simulink model "Control_model_10DOF_fin"  (R2016b)
settings: Solver=FixedStepAuto  StartTime=0.0  StopTime=10  FixedStep=0.0001  RelTol=1e-3
InitFcn:
  | Initialisation_ctr_10DOF_fin
values from neighbouring files (symbols this model uses):
  COM_Parameters = [-lpelvis/2;r2;0]    [Initialisation_ctr_10DOF_fin.m]
  DH_Parameters = [hfoot 0 ... (first row only)    [Initialisation_ctr_10DOF_fin.m]
  dTrunk = trunklbd(3)    [Initialisation_ctr_10DOF_fin.m]
  dxFootSM = dxFoot    [Initialisation_ctr_10DOF_fin.m]
  dxTrunk = 0.1    [Initialisation_ctr_10DOF_fin.m]
  Foot_Parameters = [0;-(lFoot/2-lHeel);0]    [Initialisation_ctr_10DOF_fin.m]
  HAA2HEE = [0; 0; 0.001]    [Initialisation_ctr_10DOF_fin.m]
  HEE2HFE = 0.5*[0.2; 0; 0]    [Initialisation_ctr_10DOF_fin.m]
  height_vrp = CoM_position(1)    [Initialisation_ctr_10DOF_fin.m]
  hTrunk = trunklbd(1)    [Initialisation_ctr_10DOF_fin.m]
  initial_CoM_position = R*CoM_position    [Initialisation_ctr_10DOF_fin.m]
  initial_CoM_velocity = [0;0;0]    [Initialisation_ctr_10DOF_fin.m]
  initial_left_foot = [0;0;-stance_width/2]    [Initialisation_ctr_10DOF_fin.m]
  initial_right_foot = [0;0;stance_width/2]    [Initialisation_ctr_10DOF_fin.m]
  initial_RorL = 0    [Initialisation_ctr_10DOF_fin.m]
  jointsinitial = [9;-15;6;0;0;6;-15;9]/180*pi    [Initialisation_ctr_10DOF_fin.m]
  K_DCM = 4.3*[1 0 0 ... (first row only)    [Initialisation_ctr_10DOF_fin.m]
  kD_left = mbody*[0.95 0 0 0 ... (first row only)    [Initialisation_ctr_10DOF_fin.m]
  kD_right = mbody*[0.12 0 0 0 ... (first row only)    [Initialisation_ctr_10DOF_fin.m]
  kI_left = mbody*[35 0 0 0 ... (first row only)    [Initialisation_ctr_10DOF_fin.m]
  kI_right = mbody*[38.2 0 0 0 ... (first row only)    [Initialisation_ctr_10DOF_fin.m]
  kP_left = mbody*[75 0 0 0 ... (first row only)    [Initialisation_ctr_10DOF_fin.m]
  kP_right = mbody*[5.6 0 0 0 ... (first row only)    [Initialisation_ctr_10DOF_fin.m]
  Lenght = [lShank;lThigh]    [Initialisation_ctr_10DOF_fin.m]
  lFootSM = lFoot    [Initialisation_ctr_10DOF_fin.m]
  lpelvis = wPelvis    [Initialisation_ctr_10DOF_fin.m]
  mass = mbody    (= 60)    [Initialisation_ctr_10DOF_fin.m]
  Masses = [mThigh; mShank; mTrunk]    [Initialisation_ctr_10DOF_fin.m]
  nb_step = 4    [Initialisation_ctr_10DOF_fin.m]
  nb_step_pattern = 20    [Initialisation_ctr_10DOF_fin.m]
  Pelvis_Parameters = [-lpelvis/2;hTrunk/2;0]    [Initialisation_ctr_10DOF_fin.m]
  stance_width = lpelvis    [Initialisation_ctr_10DOF_fin.m]
  stride_lenght = 0.50    (= 0.5)    [Initialisation_ctr_10DOF_fin.m]
  T_DS = time_DS    (= 0.4)    [Initialisation_ctr_10DOF_fin.m]
  T_IT = time_DS    (= 0.4)    [Initialisation_ctr_10DOF_fin.m]
  T_SS = time_swing    (= 1.6)    [Initialisation_ctr_10DOF_fin.m]
  time_DS = (time_stance-time_swing)/2    (= 0.4)    [Initialisation_ctr_10DOF_fin.m]
  time_stance = 60/100*time_stride    (= 2.4)    [Initialisation_ctr_10DOF_fin.m]
  time_step = time_stride/2    (= 2)    [Initialisation_ctr_10DOF_fin.m]
  time_swing = 40/100*time_stride    (= 1.6)    [Initialisation_ctr_10DOF_fin.m]
  validity_angle = [-20*pi/180 20*pi/180 ... (first row only)    [Initialisation_ctr_10DOF_fin.m]
  wTrunk = trunklbd(2)    [Initialisation_ctr_10DOF_fin.m]
  x4CoM = CoM_position(1)-XR4(1)    [Initialisation_ctr_10DOF_fin.m]
undefined symbols (not defined in the file or in its folder): dsegment, hFoot, l, lFoot, omega0_x, omega0_z, rho, wPelvis, X, Xp_x, Xp_z, Y, Z
undefined symbols (not defined in the file): k_grf, lShankSM, lThighSM, mShank, mThigh
libraries: nesl_utility x247, sm_lib x215, dspindex x12, FootPlacementLibrary x8, dspsigops x4, dspswit3 x1
(part 13 of 18)

== matlab function Control_model_10DOF_fin/10DoF Walker SimMechanics Model/Foot/GRF2 Toe/MATLAB Function1 ==
  data: x input; dx input; y input; dy input; z input; Fx output; dz input; Fy output; k input; Fz output
function [Fx,Fy,Fz]= fcn(x,dx,y,dy,z,dz,k)
%#codegen
% k=[5*10^4 10^4 0 10^4 0];
%k=[5*10^4 10^4 0 0 0];
% k=[0 0 0 0 0];

kp = k(1);
kv = k(2);
kpt = k(3);
kvt = k(4);
mu = k(5);

persistent prevContact;

if y>0
    Fy = 0;
    Fxz = [0;0];
    prevContact = [];
else
    if isempty(prevContact)
        prevContact = [x;z];
    end
    Current = [x;z];
    
    Fy = -kp*y-kv*dy;
%     Fxz = -kpt*(Current-prevContact)-kvt*[dx;dz];
    Fxz = -kvt*[dx;dz];
end

if Fy<0;
    Fy = 0;
%     prevContact = [];
end

mu=1;
if norm(Fxz)>mu*norm(Fy)
    Fxz = Fxz/norm(Fxz)*mu*norm(Fy);
end

Fx = Fxz(1);
Fz = Fxz(2);

== matlab function Control_model_10DOF_fin/10DoF Walker SimMechanics Model/Foot/MATLAB Function ==
  data: R_foot_pos input; TW0 output; R_foot_Rotation input; XWankleR output; Foot_Parameters parameter; DH_Parameters parameter
function [TW0,XWankleR] = fcn(R_foot_pos,R_foot_Rotation,Foot_Parameters,DH_Parameters)

% TWR=[R_foot_Rotation(1,2) R_foot_Rotation(1,1) -R_foot_Rotation(1,3) R_foot_pos(2);
%     R_foot_Rotation(2,2) R_foot_Rotation(2,1) -R_foot_Rotation(2,3) R_foot_pos(1);
%     R_foot_Rotation(3,2) R_foot_Rotation(3,1) -R_foot_Rotation(3,3) -R_foot_pos(3)
%     0 0 0 1];

xfoot=Foot_Parameters(1);
yfoot=Foot_Parameters(2);
zfoot=Foot_Parameters(3);

a0=DH_Parameters(1,1);
d1=DH_Parameters(1,2);
a1=DH_Parameters(2,1);
d2=DH_Parameters(2,2);
a2=DH_Parameters(3,1);
d3=DH_Parameters(3,2);
a3=DH_Parameters(4,1);
d4=DH_Parameters(4,2);
a4=DH_Parameters(5,1);
d5=DH_Parameters(5,2);
a5=DH_Parameters(6,1);
d6=DH_Parameters(6,2);
a6=DH_Parameters(7,1);
d7=DH_Parameters(7,2);
a7=DH_Parameters(8,1);
d8=DH_Parameters(8,2);
a8=DH_Parameters(9,1);
d9=DH_Parameters(9,2);

TWR_D=[R_foot_Rotation(1,1) R_foot_Rotation(1,2) R_foot_Rotation(1,3) R_foot_pos(1);
    R_foot_Rotation(2,1) R_foot_Rotation(2,2) R_foot_Rotation(2,3) R_foot_pos(2);
    R_foot_Rotation(3,1) R_foot_Rotation(3,2) R_foot_Rotation(3,3) R_foot_pos(3);
    0 0 0 1];

T=[0 1 0 0;
    1 0 0 0;
    0 0 -1 0;
    0 0 0 1];

TWR=TWR_D*T;

TR0=[1 0 0 xfoot;
    0 1 0 yfoot;
    0 0 1 zfoot;
    0 0 0 1];

T0ankleR=[1 0 0 a0;
    0 1 0 0;
    0 0 1 0;
    0 0 0 1];

TW0=TWR*TR0;
TWankleR=TW0*T0ankleR;

XWR=TWR(1:3,4);
XW0=TW0(1:3,4);
XWankleR=TWankleR(1:3,4);

== matlab function Control_model_10DOF_fin/10DoF Walker SimMechanics Model/Foot1/GRF1 Heel/MATLAB Function1 ==
  data: x input; dx input; y input; dy input; z input; Fx output; dz input; Fy output; k input; Fz output
function [Fx,Fy,Fz]= fcn(x,dx,y,dy,z,dz,k)
%#codegen
% k=[5*10^4 10^4 0 10^4 0];
% k=[5*10^4 10^4 0 0 0];
% k=[0 0 0 0 0];

kp = k(1);
kv = k(2);
kpt = k(3);
kvt = k(4);
mu = k(5);

persistent prevContact;

if y>0
    Fy = 0;
    Fxz = [0;0];
    prevContact = [];
else
    if isempty(prevContact)
        prevContact = [x;z];
    end
    Current = [x;z];
    
    Fy = -kp*y-kv*dy;
%     Fxz = -kpt*(Current-prevContact)-kvt*[dx;dz];
    Fxz = -kvt*[dx;dz];
end

if Fy<0
    Fy = 0;
%     prevContact = [];
end

mu=1;
if norm(Fxz)>mu*norm(Fy)
    Fxz = Fxz/norm(Fxz)*mu*norm(Fy);
end

Fx = Fxz(1);
Fz = Fxz(2);

== matlab function Control_model_10DOF_fin/10DoF Walker SimMechanics Model/Foot1/GRF1 Toe/MATLAB Function1 ==
  data: x input; dx input; y input; dy input; z input; Fx output; dz input; Fy output; k input; Fz output
function [Fx,Fy,Fz]= fcn(x,dx,y,dy,z,dz,k)
%#codegen
% k=[5*10^4 10^4 0 10^4 0];
%k=[5*10^4 10^4 0 0 0];
% k=[0 0 0 0 0];

kp = k(1);
kv = k(2);
kpt = k(3);
kvt = k(4);
mu = k(5);

persistent prevContact;

if y>0
    Fy = 0;
    Fxz = [0;0];
    prevContact = [];
else
    if isempty(prevContact)
        prevContact = [x;z];
    end
    Current = [x;z];
    
    Fy = -kp*y-kv*dy;
%     Fxz = -kpt*(Current-prevContact)-kvt*[dx;dz];
    Fxz = -kvt*[dx;dz];
end

if Fy<0;
    Fy = 0;
%     prevContact = [];
end

mu=1;
if norm(Fxz)>mu*norm(Fy)
    Fxz = Fxz/norm(Fxz)*mu*norm(Fy);
end

Fx = Fxz(1);
Fz = Fxz(2);

== matlab function Control_model_10DOF_fin/10DoF Walker SimMechanics Model/Foot1/GRF2 Heel/MATLAB Function1 ==
  data: x input; dx input; y input; dy input; z input; Fx output; dz input; Fy output; k input; Fz output
function [Fx,Fy,Fz]= fcn(x,dx,y,dy,z,dz,k)
%#codegen
% k=[5*10^4 10^4 0 10^4 0];
% k=[5*10^4 10^4 0 0 0];
% k=[0 0 0 0 0];

kp = k(1);
kv = k(2);
kpt = k(3);
kvt = k(4);
mu = k(5);

persistent prevContact;

if y>0
    Fy = 0;
    Fxz = [0;0];
    prevContact = [];
else
    if isempty(prevContact)
        prevContact = [x;z];
    end
    Current = [x;z];
    
    Fy = -kp*y-kv*dy;
%     Fxz = -kpt*(Current-prevContact)-kvt*[dx;dz];
    Fxz = -kvt*[dx;dz];
end

if Fy<0
    Fy = 0;
%     prevContact = [];
end

mu=1;
if norm(Fxz)>mu*norm(Fy)
    Fxz = Fxz/norm(Fxz)*mu*norm(Fy);
end

Fx = Fxz(1);
Fz = Fxz(2);

== matlab function Control_model_10DOF_fin/10DoF Walker SimMechanics Model/Foot1/GRF2 Toe/MATLAB Function1 ==
  data: x input; dx input; y input; dy input; z input; Fx output; dz input; Fy output; k input; Fz output
function [Fx,Fy,Fz]= fcn(x,dx,y,dy,z,dz,k)
%#codegen
% k=[5*10^4 10^4 0 10^4 0];
%k=[5*10^4 10^4 0 0 0];
% k=[0 0 0 0 0];

kp = k(1);
kv = k(2);
kpt = k(3);
kvt = k(4);
mu = k(5);

persistent prevContact;

if y>0
    Fy = 0;
    Fxz = [0;0];
    prevContact = [];
else
    if isempty(prevContact)
        prevContact = [x;z];
    end
    Current = [x;z];
    
    Fy = -kp*y-kv*dy;
%     Fxz = -kpt*(Current-prevContact)-kvt*[dx;dz];
    Fxz = -kvt*[dx;dz];
end

if Fy<0
    Fy = 0;
%     prevContact = [];
end

mu=1;
if norm(Fxz)>mu*norm(Fy)
    Fxz = Fxz/norm(Fxz)*mu*norm(Fy);
end

Fx = Fxz(1);
Fz = Fxz(2);

== matlab function Control_model_10DOF_fin/10DoF Walker SimMechanics Model/Graphic/Joint position/T->X/MATLAB Function ==
  data: XWR output; XW0 output; TWR input; TW0 input; TW1 input; XW1 output; TW2 input; TW3 input; XW2 output; TW4 input; TW5 input; TW6 input; TW7 input; TW8 input; TW9 input; TWL input; XW3 output; XW4 output; XW5 output; XW6 output; XW7 output; XW8 output; XWcom input; XW9 output; XWL output; TWthighR input; XWCoM output; TWshankR input; TWtrunk input; TWshankL input; TWthighL input; XWthighR output; XWthighL output; XWshankR output; XWshankL output; XWtrunk output
function [XWR,XW0,XW1,XW2,XW3,XW4,XW5,XW6,XW7,XW8,XW9,XWL,XWCoM,XWthighR,XWthighL,XWshankR,XWshankL,XWtrunk] = Joint_position(TWR,TW0,TW1,TW2,TW3,TW4,TW5,TW6,TW7,TW8,TW9,TWL,XWcom,TWthighR,TWshankR,TWtrunk,TWshankL,TWthighL)

XWR=TWR(1:3,4);
XW0=TW0(1:3,4);
XW1=TW1(1:3,4);
XW2=TW2(1:3,4);
XW3=TW3(1:3,4);
XW4=TW4(1:3,4);
XW5=TW5(1:3,4);
XW6=TW6(1:3,4);
XW7=TW7(1:3,4);
XW8=TW8(1:3,4);
XW9=TW9(1:3,4);
XWL=TWL(1:3,4);
XWCoM=XWcom;
XWthighR=TWthighR(1:3,4);
XWthighL=TWthighL(1:3,4);
XWshankR=TWshankR(1:3,4);
XWshankL=TWshankL(1:3,4);
XWtrunk=TWtrunk(1:3,4);

== matlab function Control_model_10DOF_fin/10DoF Walker SimMechanics Model/Graphic/Subsystem/MATLAB Function1 ==
  data: Right_foot_position input; R1 output; Left_foot_position input; lFoot parameter; dsegment parameter; r_vrp input size=3; r_DCM input size=3; R2 output; R3 output; R4 output; L1 output; L2 output; L3 output; L4 output; new_vrp output; outside output
function [R1,R2,R3,R4,L1,L2,L3,L4,new_vrp,outside] = support_polygon(Right_foot_position,Left_foot_position,lFoot,dsegment,r_vrp,r_DCM)
R1=Right_foot_position+[0;lFoot/2;dsegment/2];
R2=Right_foot_position+[0;lFoot/2;-dsegment/2];
R3=Right_foot_position+[0;-lFoot/2;-dsegment/2];
R4=Right_foot_position+[0;-lFoot/2;dsegment/2];

L1=Left_foot_position+[0;lFoot/2;dsegment/2];
L2=Left_foot_position+[0;lFoot/2;-dsegment/2];
L3=Left_foot_position+[0;-lFoot/2;-dsegment/2];
L4=Left_foot_position+[0;-lFoot/2;dsegment/2];

%Calcul affine line
a1=(L4(2)-R4(2))/(L4(3)-R4(3));
b1=R4(2)-a1*R4(3);

a2=(L2(2)-R2(2))/(L2(3)-R2(3));
b2=R2(2)-a2*R2(3);

a3=(r_vrp(2)-r_DCM(2))/(r_vrp(3)-r_DCM(3));
b3=r_DCM(2)-a3*r_DCM(3);

%Check if outside support polygon (1=outside,0=indside)
outside=0;



if ((r_vrp(2)<R3(2)) || (r_vrp(2)>L1(2)) || (r_vrp(3)<R3(3)) || (r_vrp(3)>L1(3)))
    outside=1;
elseif (r_vrp(2)<a1*r_vrp(3)+b1) || (r_vrp(2)>a2*r_vrp(3)+b2)
        outside=1;
end

% if outside ==1
% else
%     new_vrp=r_vrp;
% end


new_vrp=r_vrp;
if outside==1
    if r_vrp(3)<=R3(3)
        new_vrp(3)=R3(3);
        new_vrp(2)=a3*new_vrp(3)+b3;
        if new_vrp(2)<R3(2)
            new_vrp(2)=R3(2);
            new_vrp(3)=(new_vrp(2)-b3)/a3;
            if new_vrp(3)<R3(3)
                new_vrp(2)=R3(2);
                new_vrp(3)=R3(3);
            elseif new_vrp(2)<R4(2)
                new_vrp(2)=R4(2);
                new_vrp(3)=R4(3);
            end      
        elseif new_vrp(2)>R2(2)
            new_vrp(3)=(b2-b1)/(a1-a2);
            new_vrp(2)=a3*new_vrp(3)+b3;
            if new_vrp(3)<R2(3)
                new_vrp(2)=R2(2);
                new_vrp(3)=R2(3);
            end
        end
    elseif r_vrp(3)>=L1(3)
        new_vrp(3)=L1(3);
        new_vrp(2)=a3*new_vrp(3)+b3;
        if new_vrp(2)<L4(2)
            new_vrp(3)=(b3-b1)/(a3-a1);
            new_vrp(2)=a3*new_vrp(3)+b3;
            if new_vrp(2)<L4(2)
                new_vrp(2)=L4(2);
                new_vrp(3)=L4(3);
            end
        elseif new_vrp(2)>L1(2)
            new_vrp(2)=L1(2);
            new_vrp(3)=(new_vrp(2)-b3)/a3;
            if new_vrp(3)>L1(3)
                new_vrp(2)=L1(2);
                new_vrp(3)=L1(3);
            elseif new_vrp(3)<L2(3)
                new_vrp(2)=L2(2);
                new_vrp(3)=L2(3);
            end
                
        end
        
    elseif r_vrp(2)<=R3(2)
        new_vrp(2)=R3(2);
        new_vrp(3)=(new_vrp(2)-b3)/a3;
        if new_vrp(3)<R3(3)
            new_vrp(2)=R3(2);
            new_vrp(3)=R3(3);
        elseif new_vrp(3)>R4(3)
                new_vrp(3)=(b3-b1)/(a3-a1);
                new_vrp(2)=a3*new_vrp(3)+b3;
                if new_vrp(3)<R4(3)
                    new_vrp(2)=R4(2);
                    new_vrp(3)=R4(3);
                elseif new_vrp(3)>L4(3)
                    new_vrp(2)=L4(2);
                    new_vrp(3)=L4(3);
                end
        end
    elseif r_vrp(2)>=L1(2)
        new_vrp(2)=L1(2);
        new_vrp(3)=(new_vrp(2)-b3)/a3;
        if new_vrp(3)>L1(3)
            new_vrp(2)=L1(2);
            new_vrp(3)=L1(3);
        elseif new_vrp(3)<L2(3)
            new_vrp(3)=(b2-b3)/(a2-a3);
            new_vrp(2)=a3*new_vrp(3)+b3;
            if new_vrp(3)>L2(3)
                new_vrp(2)=L2(2);
                new_vrp(3)=L2(3);
            elseif new_vrp(3)<R2(3)
                new_vrp(2)=R2(2);
                new_vrp(3)=R3(2);
            end
        end
    end
end

== matlab function Control_model_10DOF_fin/10DoF Walker SimMechanics Model/Graphic/Subsystem/MATLAB Function2 ==
  data: Right_foot_position input; R1 output; Left_foot_position input; lFoot parameter; dsegment parameter; r_vrp input size=3; r_DCM input size=3; R2 output; R3 output; R4 output; L1 output; L2 output; L3 output; L4 output; new_vrp output; outside output; cas output
function [R1,R2,R3,R4,L1,L2,L3,L4,new_vrp,outside,cas] = support_polygon(Right_foot_position,Left_foot_position,lFoot,dsegment,r_vrp,r_DCM)
R1=Right_foot_position+[0;lFoot/2;dsegment/2];
R2=Right_foot_position+[0;lFoot/2;-dsegment/2];
R3=Right_foot_position+[0;-lFoot/2;-dsegment/2];
R4=Right_foot_position+[0;-lFoot/2;dsegment/2];

L1=Left_foot_position+[0;lFoot/2;dsegment/2];
L2=Left_foot_position+[0;lFoot/2;-dsegment/2];
L3=Left_foot_position+[0;-lFoot/2;-dsegment/2];
L4=Left_foot_position+[0;-lFoot/2;dsegment/2];

%Calcul affine line

a1=(L1(2)-R1(2))/(L1(3)-R1(3));
b1=R1(2)-a1*R1(3);

a2=(L2(2)-R2(2))/(L2(3)-R2(3));
b2=R2(2)-a2*R2(3);

a3=(L3(2)-R3(2))/(L3(3)-R3(3));
b3=R3(2)-a3*R3(3);

a4=(L4(2)-R4(2))/(L4(3)-R4(3));
b4=R4(2)-a4*R4(3);

a5=(r_vrp(2)-r_DCM(2))/(r_vrp(3)-r_DCM(3));
b5=r_DCM(2)-a5*r_DCM(3);


%Check if outside support polygon (1=outside,0=indside)
outside=0;






% if outside ==1
% else
%     new_vrp=r_vrp;
% end

point=r_vrp;
point(3)=(b5-b4)/(a5-a4);
point(2)=a5*r_vrp(3)+b5;

cas=0;

new_vrp=r_vrp;

%% Right

if ((r_vrp(2)<R3(2)) || (r_vrp(2)>L1(2)) || (r_vrp(3)<R3(3)) || (r_vrp(3)>L1(3)))
    outside=1;
elseif (r_vrp(2)<a4*r_vrp(3)+b4) || (r_vrp(2)>a2*r_vrp(3)+b2)
        outside=1;
end

if outside==1
    if r_vrp(3)<=R3(3)
        new_vrp(3)=R3(3);
        new_vrp(2)=a5*new_vrp(3)+b5;
        cas=1;
        if new_vrp(2)<R3(2)
            new_vrp(2)=R3(2);
            new_vrp(3)=(new_vrp(2)-b5)/a5;
            cas=2;
            if new_vrp(3)<R3(3)
                new_vrp(2)=R3(2);
                new_vrp(3)=R3(3);
                cas=3;
            elseif new_vrp(2)<R4(2)
                new_vrp(2)=R4(2);
                new_vrp(3)=R4(3);
                cas=4;
            end      
        elseif new_vrp(2)>R2(2)
            new_vrp(3)=(b2-b5)/(a5-a2);
            new_vrp(2)=a5*new_vrp(3)+b5;
            cas=5;
            if new_vrp(3)<R2(3)
                new_vrp(2)=R2(2);
                new_vrp(3)=R2(3);
                cas=6;
            end
        end
    elseif r_vrp(3)>=L1(3)
        new_vrp(3)=L1(3);
        new_vrp(2)=a5*new_vrp(3)+b5;
        cas=7;
        if new_vrp(2)<L4(2)
            new_vrp(3)=(b5-b4)/(a4-a5);
            new_vrp(2)=a5*new_vrp(3)+b5;
            cas=8;
            if new_vrp(3)>L4(3)
                new_vrp(2)=L4(2);
                new_vrp(3)=L4(3);
                cas=9;
            elseif new_vrp(3)<R4(3)
                new_vrp(2)=R4(2);
                new_vrp(3)=R4(3);
                cas=10;
            end
        elseif new_vrp(2)>L1(2)
            new_vrp(2)=L1(2);
            new_vrp(3)=(new_vrp(2)-b5)/a5;
            cas=11;
            if new_vrp(3)>L1(3)
                new_vrp(2)=L1(2);
                new_vrp(3)=L1(3);
                cas=12;
            elseif new_vrp(3)<L2(3)
                new_vrp(2)=L2(2);
                new_vrp(3)=L2(3);
                cas=13;
            end
                
        end
        
    elseif r_vrp(2)<=R3(2)
        new_vrp(2)=R3(2);
        new_vrp(3)=(new_vrp(2)-b5)/a5;
        cas=14;
        if new_vrp(3)<R3(3)
            new_vrp(2)=R3(2);
            new_vrp(3)=R3(3);
            cas=15;
        elseif new_vrp(3)>R4(3)
                new_vrp(3)=(b5-b4)/(a4-a5);
                new_vrp(2)=a5*new_vrp(3)+b5;
                cas=16;
                if new_vrp(3)<R4(3)
                    new_vrp(2)=R4(2);
                    new_vrp(3)=R4(3);
                    cas=17;
                elseif new_vrp(3)>L4(3)
                    new_vrp(2)=L4(2);
                    new_vrp(3)=L4(3);
                    cas=18;
                end
        end
    elseif r_vrp(2)>=L1(2)
        new_vrp(2)=L1(2);
        new_vrp(3)=(new_vrp(2)-b5)/a5;
        cas=19;
        if new_vrp(3)>L1(3)
            new_vrp(2)=L1(2);
            new_vrp(3)=L1(3);
            cas=20;
        elseif new_vrp(3)<L2(3)
            new_vrp(3)=(b2-b5)/(a5-a2);
            new_vrp(2)=a5*new_vrp(3)+b5;
            cas=21;
            if new_vrp(3)>L2(3)
                new_vrp(2)=L2(2);
                new_vrp(3)=L2(3);
                cas=22;
            elseif new_vrp(3)<R2(3)
                new_vrp(2)=R2(2);
                new_vrp(3)=R3(2);
                cas=23;
            end
        end
    elseif (r_vrp(2)<a4*r_vrp(3)+b4)
        new_vrp(3)=(b4-b5)/(a5-a4);
        new_vrp(2)=a5*new_vrp(3)+b5;
        cas=24;
        if new_vrp(3)<R4(3)
            new_vrp(2)=R4(2);
            new_vrp(3)=R4(3);
            cas=25;
        elseif new_vrp(2)>L4
            new_vrp(2)=L4(2);
            new_vrp(3)=L4(3);
            cas=26;
        end
    elseif (r_vrp(2)>a2*r_vrp(3)+b2)
        new_vrp(3)=(b5-b2)/(a2-a5);
        new_vrp(2)=a5*new_vrp(3)+b5;
        cas=27;
        if new_vrp(3)<R2(3)
            new_vrp(2)=R2(2);
            new_vrp(3)=R2(3);
            cas=28;
        elseif new_vrp(3)>L2(3)
            new_vrp(2)=L2(3);
            new_vrp(3)=L2(3);
            cas=29;
        end
    end
end

%% Left

% if ((r_vrp(2)<L4(2)) || (r_vrp(2)>R2(2)) || (r_vrp(3)<R2(3)) || (r_vrp(3)>L4(3)))
%     outside=1;
% elseif (r_vrp(2)<a3*r_vrp(3)+b3) || (r_vrp(2)>a1*r_vrp(3)+b1)
%         outside=1;
% end

% new_vrp=r_vrp;

% if outside==1
%     if r_vrp(3)>L4(3)
%         new_vrp(3)=L4(3);
%         new_vrp(2)=a5*new_vrp(3)+b5;
%         if new_vrp(2)<L4(2)
%             new_vrp(2)=L4(2);
%             new_vrp(3)=(new_vrp(2)-b5)/a5;
%             if new_vrp(3)>L4(3)
%                 new_vrp(2)=L4(2);
%                 new_vrp(3)=L4(3);
%             elseif new_vrp(3)<L3(3)
%                 new_vrp(2)=L3(2);
%                 new_vrp(3)=L3(3);
%             end
%         elseif new_vrp(2)>L1(2)
%             new_vrp(3)=(b1-b5)/(a1-a5);
%             new_vrp(2)=a5*new_vrp(3)+b5;
%             if new_vrp(3)>L1(3)
%                 new_vrp(2)=L1(2);
%                 new_vrp(3)=L1(3);
%             elseif new_vrp(2)<R1(2)
%                 new_vrp(2)=R1(2);
%                 new_vrp(3)=R1(3);
%             end
%         end
%     elseif r_vrp(3)<R2(3)
%         new_vrp(3)=R2(3);
%         new_vrp(2)=a5*new_vrp(3)+b5;
%         if new_vrp(2)>R2(2)
%             new_vrp(2)=R2(2);
%             new_vrp(3)=(new_vrp(2)-b5)/a5;
%             if new_vrp(3)<R2(3)
%                 new_vrp(2)=R2(2);
%                 new_vrp(3)=R2(3);
%             elseif new_vrp(3)>R1(3)
%                 new_vrp(2)=R1(2);
%                 new_vrp(3)=R1(3);
%             end
%         elseif new_vrp(2)<R3(2)
%             new_vrp(3)=(b3-b5)/(a3-a5);
%             new_vrp(2)=a5*new_vrp(3)+b5;
%             if new_vrp(3)<R3(3)
%                 new_vrp(2)=R3(2);
%                 new_vrp(3)=R3(3);
%             elseif new_vrp(3)>L3(3)
%                 new_vrp(2)=L3(2);
%                 new_vrp(3)=L3(3);
%             end
%         end
%     elseif r_vrp(2)<L4(2)
%         new_vrp(2)=L4(2);
%         new_vrp(3)=(new_vrp(2)-b5)/a5;
%         if new_vrp(3)>L4(3)
%             new_vrp(3)=L4(3);
%             new_vrp(2)=a5*new_vrp(3)+b5;
%             if new_vrp(2)<L4(2)
%                 new_vrp(2)=L4(2);
%                 new_vrp(3)=L4(3);
%             elseif new_vrp(2)>L1(2)
%                 new_vrp(2)=L1(2);
%                 new_vrp(3)=L1(3);
%             end
%         elseif new_vrp(3)<L3(3)
%             new_vrp(3)=(b3-b5)/(a3-a5);
%             new_vrp(2)=a5*new_vrp(3)+b5;
%             if new_vrp(3)>L3(3)
%                 new_vrp(2)=L3(2);
%                 new_vrp(3)=L3(3);
%             elseif new_vrp(3)<R3(3)
%                 new_vrp(2)=R3(2);
%                 new_vrp(3)=R3(3);
%             end
%         end
%     elseif r_vrp(2)>R2(2)
%         new_vrp(2)=R2(2);
%         new_vrp(3)=(new_vrp(2)-b5)/a5;
%         if new_vrp(3)<R2(3)
%             new_vrp(3)=R2(3);
%             new_vrp(2)=a5*new_vrp(3)+b5;
%             if new_vrp(2)<R3(2)
%                 new_vrp(2)=R3(2);
%                 new_vrp(3)=R3(3);
%             elseif new_vrp(2)>R2(2)
%                    new_vrp(2)=R2(2);
%                    new_vrp(3)=R2(3);
%             end
%         elseif new_vrp(3)>R1(3)
%             new_vrp(3)=(b1-b5)/(a1-a5);
%             new_vrp(2)=a5*new_vrp(3)+b5;
%             if new_vrp(3)<R1(3)
%                 new_vrp(2)=R1(2);
%                 new_vrp(3)=R1(3);
%             elseif new_vrp(3)>L1(3)
%                 new_vrp(2)=L1(2);
%                 new_vrp(3)=L1(3);
%             end
%         end
%     end
% end

== matlab function Control_model_10DOF_fin/10DoF Walker SimMechanics Model/Graphic/Subsystem/MATLAB Function3 ==
  data: TWR input; R1 output; Left_foot_position input; lFoot parameter; dsegment parameter; r_vrp_W input size=3; r_DCM_W input size=3; R2 output; R3 output; R4 output; L1 output; L2 output; L3 output; L4 output; new_vrp output; outside output
function [R1,R2,R3,R4,L1,L2,L3,L4,new_vrp,outside]  = support_polygon(TWR,Left_foot_position,lFoot,dsegment,r_vrp_W,r_DCM_W)

XWR=TWR(1:3,4);
RWR=TWR(1:3,1:3);

R1W=XWR+RWR*[0;lFoot/2;dsegment/2];
R1W(2)=0;
R2W=XWR+RWR*[0;lFoot/2;-dsegment/2];
R2W(2)=0;
R3W=XWR+RWR*[0;-lFoot/2;-dsegment/2];
R3W(2)=0;
R4W=XWR+RWR*[0;-lFoot/2;dsegment/2];
R4W(2)=0;

L1W=Left_foot_position+RWR*[0;lFoot/2;dsegment/2];
L1W(2)=0;
L2W=Left_foot_position+RWR*[0;lFoot/2;-dsegment/2];
L2W(2)=0;
L3W=Left_foot_position+RWR*[0;-lFoot/2;-dsegment/2];
L3W(2)=0;
L4W=Left_foot_position+RWR*[0;-lFoot/2;dsegment/2];
L4W(2)=0;

R1=RWR*(R1W-XWR);
R2=RWR*(R2W-XWR);
R3=RWR*(R3W-XWR);
R4=RWR*(R4W-XWR);

L1=RWR*(L1W-XWR);
L2=RWR*(L2W-XWR);
L3=RWR*(L3W-XWR);
L4=RWR*(L4W-XWR);

save=r_vrp_W(2);
r_vrp_W(2)=0;
r_vrp=RWR*(r_vrp_W-XWR);
r_DCM_W(2)=0;
r_DCM=RWR*(r_DCM_W-XWR);

%Calcul affine line
a1=(L1(2)-R1(2))/(L1(3)-R1(3));
b1=R1(2)-a1*R1(3);

a2=(L2(2)-R2(2))/(L2(3)-R2(3));
b2=R2(2)-a2*R2(3);

a3=(L3(2)-R3(2))/(L3(3)-R3(3));
b3=R3(2)-a3*R3(3);

a4=(L4(2)-R4(2))/(L4(3)-R4(3));
b4=R4(2)-a4*R4(3);

a5=(r_vrp(2)-r_DCM(2))/(r_vrp(3)-r_DCM(3));
b5=r_DCM(2)-a5*r_DCM(3);

outside=0;

if ((r_vrp(2)>R1(2)) || (r_vrp(2)<R3(2)) || (r_vrp(3)>R1(3)) || (r_vrp(3)<R3(3)))
    outside=1;
end

new_vrp=r_vrp;

if outside==1
    if r_vrp(2)<R3(2)
        new_vrp(2)=R3(2);
        new_vrp(3)=(new_vrp(2)-b5)/a5;
        if new_vrp(3)<R3(3)
            new_vrp(3)=R3(3);
            new_vrp(2)=a5*new_vrp(3)+b5;
            if new_vrp(2)<R3(2)
                new_vrp(2)=R3(2);
                new_vrp(3)=R3(3);
            elseif new_vrp(2)>R2(2)
                new_vrp(2)=R2(2);
                new_vrp(3)=R2(3);
            end
        elseif new_vrp(3)>R4(3)
            new_vrp(3)=R4(3);
            new_vrp(2)=a5*new_vrp(3)+b5;
            if new_vrp(2)<R4(2)
                new_vrp(2)=R4(2);
                new_vrp(3)=R4(3);
            elseif new_vrp(2)>R1(2)
                new_vrp(2)=R1(2);
                new_vrp(3)=R1(3);
            end
        end
    elseif r_vrp(2)>R1(2)
        new_vrp(2)=R1(2);
        new_vrp(3)=(new_vrp(2)-b5)/a5;
        if new_vrp(3)>R1(3)
            new_vrp(3)=R1(3);
            new_vrp(2)=a5*new_vrp(3)+b5;
            if new_vrp(2)>R1(2)
                new_vrp(2)=R1(2);
                new_vrp(3)=R1(3);
            elseif new_vrp(2)<R4(2)
                new_vrp(2)=R4(2);
                new_vrp(3)=R4(3);
            end
        elseif new_vrp(3)<R2(3)
            new_vrp(3)=R2(3);
            new_vrp(2)=a5*new_vrp(3)+b5;
            if new_vrp(2)>R2(2)
                new_vrp(2)=R2(2);
                new_vrp(3)=R2(3);
            elseif new_vrp(2)<R3(2)
                new_vrp(2)=R3(2);
                new_vrp(3)=R3(3);
            end
        end
    elseif r_vrp(3)<R3(3)
        new_vrp(3)=R3(3);
        new_vrp(2)=a5*new_vrp(3)+b5;
        if new_vrp(2)>R2(2)
            new_vrp(2)=R2(2);
            new_vrp(3)=(new_vrp(2)-b5)/a5;
            if new_vrp(3)<R2(3)
                new_vrp(2)=R2(2);
                new_vrp(3)=R2(3);
            elseif new_vrp(3)>R1(3)
                new_vrp(2)=R1(2);
                new_vrp(3)=R1(3);
            end
        elseif new_vrp(2)<R3(2)
            new_vrp(2)=R3(2);
            new_vrp(3)=(new_vrp(2)-b5)/a5;
            if new_vrp(3)<R3(3)
                new_vrp(2)=R3(2);
                new_vrp(3)=R3(3);
            elseif new_vrp(3)>R4(3)
                new_vrp(2)=R4(2);
                new_vrp(3)=R4(3);
            end 
        end
    elseif r_vrp(3)>R1(3)
        new_vrp(3)=R1(3);
        new_vrp(2)=a5*new_vrp(3)+b5;
        if new_vrp(2)>R1(2)
            new_vrp(2)=R1(2);
            new_vrp(3)=(new_vrp(2)-b5)/a5;
            if new_vrp(3)<R2(3)
                new_vrp(2)=R2(2);
                new_vrp(3)=R2(3);
            elseif new_vrp(3)>R1(3)
                new_vrp(2)=R1(2);
                new_vrp(3)=R1(3);
            end 
        elseif new_vrp(2)<R4(2)
            new_vrp(2)=R4(2);
            new_vrp(3)=(new_vrp(2)-b5)/a5;
            if new_vrp(3)<R3(3)
                new_vrp(2)=R3(2);
                new_vrp(3)=R3(3);
            elseif new_vrp(3)>R4(3)
                new_vrp(2)=R4(2);
                new_vrp(3)=R4(3);
            end 
        end
    end 
end

new_vrp=RWR.'*new_vrp+XWR;
new_vrp(2)=save;


R1=RWR.'*R1+XWR;
R2=RWR.'*R2+XWR;
R3=RWR.'*R3+XWR;
R4=RWR.'*R4+XWR;

L1=RWR.'*L1+XWR;
L2=RWR.'*L2+XWR;
L3=RWR.'*L3+XWR;
L4=RWR.'*L4+XWR;

== matlab function Control_model_10DOF_fin/10DoF Walker SimMechanics Model/Graphic/Subsystem/MATLAB Function4 ==
  data: TWR input; R1 output; Left_foot_position input; lFoot parameter; dsegment parameter; r_vrp_W input size=3; r_DCM_W input size=3; R2 output; R3 output; R4 output; L1 output; L2 output; L3 output; L4 output; new_vrp output
function [R1,R2,R3,R4,L1,L2,L3,L4,new_vrp]  = support_polygon(TWR,Left_foot_position,lFoot,dsegment,r_vrp_W,r_DCM_W)

XWR=TWR(1:3,4);
RWR=TWR(1:3,1:3);

R1W=XWR+RWR*[0;lFoot/2;dsegment/2];
R2W=XWR+RWR*[0;lFoot/2;-dsegment/2];
R3W=XWR+RWR*[0;-lFoot/2;-dsegment/2];
R4W=XWR+RWR*[0;-lFoot/2;dsegment/2];

L1W=Left_foot_position+RWR*[0;lFoot/2;dsegment/2];
L2W=Left_foot_position+RWR*[0;lFoot/2;-dsegment/2];
L3W=Left_foot_position+RWR*[0;-lFoot/2;-dsegment/2];
L4W=Left_foot_position+RWR*[0;-lFoot/2;dsegment/2];

R1=RWR*(R1W-XWR);
R2=RWR*(R2W-XWR);
R3=RWR*(R3W-XWR);
R4=RWR*(R4W-XWR);

L1=RWR*(L1W-XWR);
L2=RWR*(L2W-XWR);
L3=RWR*(L3W-XWR);
L4=RWR*(L4W-XWR);

new_vrp=0;








R1=RWR.'*R1+XWR;
R2=RWR.'*R2+XWR;
R3=RWR.'*R3+XWR;
R4=RWR.'*R4+XWR;

L1=RWR.'*L1+XWR;
L2=RWR.'*L2+XWR;
L3=RWR.'*L3+XWR;
L4=RWR.'*L4+XWR;



r_vrp=RWR*(r_vrp_W-XWR);
r_DCM=RWR*(r_DCM_W-XWR);

== matlab function Control_model_10DOF_fin/10DoF Walker SimMechanics Model/Graphic/Subsystem/MATLAB Function5 ==
  data: TWR input; R1 output; Left_foot_position input; lFoot parameter; dsegment parameter; r_vrp_W input size=3; r_DCM_W input size=3; R2 output; R3 output; R4 output; L1 output; L2 output; L3 output; L4 output; new_vrp_W output; outside output
function [R1,R2,R3,R4,L1,L2,L3,L4,new_vrp_W,outside]  = support_polygon(TWR,Left_foot_position,lFoot,dsegment,r_vrp_W,r_DCM_W)

XWR=TWR(1:3,4);
RWR=TWR(1:3,1:3);

R1W=XWR+RWR*[0;lFoot/2;dsegment/2];
R2W=XWR+RWR*[0;lFoot/2;-dsegment/2];
R3W=XWR+RWR*[0;-lFoot/2;-dsegment/2];
R4W=XWR+RWR*[0;-lFoot/2;dsegment/2];

L1W=Left_foot_position+RWR*[0;lFoot/2;dsegment/2];
L2W=Left_foot_position+RWR*[0;lFoot/2;-dsegment/2];
L3W=Left_foot_position+RWR*[0;-lFoot/2;-dsegment/2];
L4W=Left_foot_position+RWR*[0;-lFoot/2;dsegment/2];

% R1=RWR*(R1W-XWR);
% R2=RWR*(R2W-XWR);
% R3=RWR*(R3W-XWR);
% R4=RWR*(R4W-XWR);

% R1=[0;lFoot/2;dsegment/2];
% R2=[0;lFoot/2;-dsegment/2];
% R3=[0;-lFoot/2;-dsegment/2];
% R4=[0;-lFoot/2;dsegment/2];

R1=[0;lFoot/3;dsegment/3];
R2=[0;lFoot/3;-dsegment/3];
R3=[0;-lFoot/3;-dsegment/3];
R4=[0;-lFoot/3;dsegment/3];

% L1=RWR*(L1W-XWR);
% L2=RWR*(L2W-XWR);
% L3=RWR*(L3W-XWR);
% L4=RWR*(L4W-XWR);

% L1=RWR.'*(Left_foot_position-XWR)+[0;lFoot/2;dsegment/2];
% L2=RWR.'*(Left_foot_position-XWR)+[0;lFoot/2;-dsegment/2];
% L3=RWR.'*(Left_foot_position-XWR)+[0;-lFoot/2;-dsegment/2];
% L4=RWR.'*(Left_foot_position-XWR)+[0;-lFoot/2;dsegment/2];

L1=RWR.'*(Left_foot_position-XWR)+[0;lFoot/3;dsegment/3];
L2=RWR.'*(Left_foot_position-XWR)+[0;lFoot/3;-dsegment/3];
L3=RWR.'*(Left_foot_position-XWR)+[0;-lFoot/3;-dsegment/3];
L4=RWR.'*(Left_foot_position-XWR)+[0;-lFoot/3;dsegment/3];


r_vrp=RWR.'*(r_vrp_W-XWR);
r_DCM=RWR.'*(r_DCM_W-XWR);

%Calcul affine line
a1=(L1(2)-R1(2))/(L1(3)-R1(3));
b1=R1(2)-a1*R1(3);

a2=(L2(2)-R2(2))/(L2(3)-R2(3));
b2=R2(2)-a2*R2(3);

a3=(L3(2)-R3(2))/(L3(3)-R3(3));
b3=R3(2)-a3*R3(3);

a4=(L4(2)-R4(2))/(L4(3)-R4(3));
b4=R4(2)-a4*R4(3);

a5=(r_vrp(2)-r_DCM(2))/(r_vrp(3)-r_DCM(3));
b5=r_DCM(2)-a5*r_DCM(3);


outside=0;

if ((r_vrp(2)>R1(2)) || (r_vrp(2)<R3(2)) || (r_vrp(3)>R1(3)) || (r_vrp(3)<R3(3)))
    outside=1;
    if r_vrp(2)<(a4*r_vrp(3)+b4) || r_vrp(2)>(a2*r_vrp(3)+b2)
        outside=1;
    end
end

new_vrp=r_vrp;

if outside==1
    if r_vrp(2)<R3(2)
        new_vrp(2)=R3(2);
        new_vrp(3)=(new_vrp(2)-b5)/a5;
        if new_vrp(3)<R3(3)
            new_vrp(3)=R3(3);
            new_vrp(2)=a5*new_vrp(3)+b5;
            if new_vrp(2)<R3(2)
                new_vrp(2)=R3(2);
                new_vrp(3)=R3(3);
            elseif new_vrp(2)>R2(2)
                new_vrp(2)=R2(2);
                new_vrp(3)=R2(3);
            end
        elseif new_vrp(3)>R4(3)
            new_vrp(3)=R4(3);
            new_vrp(2)=a5*new_vrp(3)+b5;
            if new_vrp(2)<R4(2)
                new_vrp(2)=R4(2);
                new_vrp(3)=R4(3);
            elseif new_vrp(2)>R1(2)
                new_vrp(2)=R1(2);
                new_vrp(3)=R1(3);
            end
        end
    elseif r_vrp(2)>R1(2)
        new_vrp(2)=R1(2);
        new_vrp(3)=(new_vrp(2)-b5)/a5;
        if new_vrp(3)>R1(3)
            new_vrp(3)=R1(3);
            new_vrp(2)=a5*new_vrp(3)+b5;
            if new_vrp(2)>R1(2)
                new_vrp(2)=R1(2);
                new_vrp(3)=R1(3);
            elseif new_vrp(2)<R4(2)
                new_vrp(2)=R4(2);
                new_vrp(3)=R4(3);
            end
        elseif new_vrp(3)<R2(3)
            new_vrp(3)=R2(3);
            new_vrp(2)=a5*new_vrp(3)+b5;
            if new_vrp(2)>R2(2)
                new_vrp(2)=R2(2);
                new_vrp(3)=R2(3);
            elseif new_vrp(2)<R3(2)
                new_vrp(2)=R3(2);
                new_vrp(3)=R3(3);
            end
        end
    elseif r_vrp(3)<R3(3)
        new_vrp(3)=R3(3);
        new_vrp(2)=a5*new_vrp(3)+b5;
        if new_vrp(2)>R2(2)
            new_vrp(2)=R2(2);
            new_vrp(3)=(new_vrp(2)-b5)/a5;
            if new_vrp(3)<R2(3)
                new_vrp(2)=R2(2);
                new_vrp(3)=R2(3);
            elseif new_vrp(3)>R1(3)
                new_vrp(2)=R1(2);
                new_vrp(3)=R1(3);
            end
        elseif new_vrp(2)<R3(2)
            new_vrp(2)=R3(2);
            new_vrp(3)=(new_vrp(2)-b5)/a5;
            if new_vrp(3)<R3(3)
                new_vrp(2)=R3(2);
                new_vrp(3)=R3(3);
            elseif new_vrp(3)>R4(3)
                new_vrp(2)=R4(2);
                new_vrp(3)=R4(3);
            end 
        end
    elseif r_vrp(3)>R1(3)
        new_vrp(3)=R1(3);
        new_vrp(2)=a5*new_vrp(3)+b5;
        if new_vrp(2)>R1(2)
            new_vrp(2)=R1(2);
            new_vrp(3)=(new_vrp(2)-b5)/a5;
            if new_vrp(3)<R2(3)
                new_vrp(2)=R2(2);
                new_vrp(3)=R2(3);
            elseif new_vrp(3)>R1(3)
                new_vrp(2)=R1(2);
                new_vrp(3)=R1(3);
            end 
        elseif new_vrp(2)<R4(2)
            new_vrp(2)=R4(2);
            new_vrp(3)=(new_vrp(2)-b5)/a5;
            if new_vrp(3)<R3(3)
                new_vrp(2)=R3(2);
                new_vrp(3)=R3(3);
            elseif new_vrp(3)>R4(3)
                new_vrp(2)=R4(2);
                new_vrp(3)=R4(3);
            end 
        end
    end 
end

new_vrp_W=RWR*new_vrp+XWR;





% R1=RWR.'*R1+XWR;
% R2=RWR.'*R2+XWR;
% R3=RWR.'*R3+XWR;
% R4=RWR.'*R4+XWR;
% 
% L1=RWR.'*L1+XWR;
% L2=RWR.'*L2+XWR;
% L3=RWR.'*L3+XWR;
% L4=RWR.'*L4+XWR;

R1=RWR*R1+XWR;
R2=RWR*R2+XWR;
R3=RWR*R3+XWR;
R4=RWR*R4+XWR;

L1=RWR*L1+XWR;
L2=RWR*L2+XWR;
L3=RWR*L3+XWR;
L4=RWR*L4+XWR;

== matlab function Control_model_10DOF_fin/10DoF Walker SimMechanics Model/Graphic/Subsystem/MATLAB Function6 ==
  data: TWR input; R1 output; Left_foot_position input; lFoot parameter; dsegment parameter; r_vrp_W input size=3; r_DCM_W input size=3; R2 output; R3 output; R4 output; L1 output; L2 output; L3 output; L4 output; new_vrp_W output; outside output
function [R1,R2,R3,R4,L1,L2,L3,L4,new_vrp_W,outside]  = support_polygon(TWR,Left_foot_position,lFoot,dsegment,r_vrp_W,r_DCM_W)

XWR=TWR(1:3,4);
RWR=TWR(1:3,1:3);

R1W=XWR+RWR*[0;lFoot/2;dsegment/2];
R2W=XWR+RWR*[0;lFoot/2;-dsegment/2];
R3W=XWR+RWR*[0;-lFoot/2;-dsegment/2];
R4W=XWR+RWR*[0;-lFoot/2;dsegment/2];

L1W=Left_foot_position+RWR*[0;lFoot/2;dsegment/2];
L2W=Left_foot_position+RWR*[0;lFoot/2;-dsegment/2];
L3W=Left_foot_position+RWR*[0;-lFoot/2;-dsegment/2];
L4W=Left_foot_position+RWR*[0;-lFoot/2;dsegment/2];

% R1=RWR*(R1W-XWR);
% R2=RWR*(R2W-XWR);
% R3=RWR*(R3W-XWR);
% R4=RWR*(R4W-XWR);
R1=[0;lFoot/2;dsegment/2];
R2=[0;lFoot/2;-dsegment/2];
R3=[0;-lFoot/2;-dsegment/2];
R4=[0;-lFoot/2;dsegment/2];

% L1=RWR*(L1W-XWR);
% L2=RWR*(L2W-XWR);
% L3=RWR*(L3W-XWR);
% L4=RWR*(L4W-XWR);

L1=RWR.'*(Left_foot_position-XWR)+[0;lFoot/2;dsegment/2];
L2=RWR.'*(Left_foot_position-XWR)+[0;lFoot/2;-dsegment/2];
L3=RWR.'*(Left_foot_position-XWR)+[0;-lFoot/2;-dsegment/2];
L4=RWR.'*(Left_foot_position-XWR)+[0;-lFoot/2;dsegment/2];

r_vrp=RWR.'*(r_vrp_W-XWR);
r_DCM=RWR.'*(r_DCM_W-XWR);

%Calcul affine line
a1=(L1(2)-R1(2))/(L1(3)-R1(3));
b1=R1(2)-a1*R1(3);

a2=(L2(2)-R2(2))/(L2(3)-R2(3));
b2=R2(2)-a2*R2(3);

a3=(L3(2)-R3(2))/(L3(3)-R3(3));
b3=R3(2)-a3*R3(3);

a4=(L4(2)-R4(2))/(L4(3)-R4(3));
b4=R4(2)-a4*R4(3);

a5=(r_vrp(2)-r_DCM(2))/(r_vrp(3)-r_DCM(3));
b5=r_DCM(2)-a5*r_DCM(3);

outside=0;

if ((r_vrp(2)>R1(2)) || (r_vrp(2)<R3(2)) || (r_vrp(3)>R1(3)) || (r_vrp(3)<R3(3)))
    outside=1;
end

new_vrp=r_vrp;

if outside==1
    if r_vrp(2)<R3(2)
        new_vrp(2)=R3(2);
        new_vrp(3)=(new_vrp(2)-b5)/a5;
        if new_vrp(3)<R3(3)
            new_vrp(3)=R3(3);
            new_vrp(2)=a5*new_vrp(3)+b5;
            if new_vrp(2)<R3(2)
                new_vrp(2)=R3(2);
                new_vrp(3)=R3(3);
            elseif new_vrp(2)>R2(2)
                new_vrp(2)=R2(2);
                new_vrp(3)=R2(3);
            end
        elseif new_vrp(3)>R4(3)
            new_vrp(3)=R4(3);
            new_vrp(2)=a5*new_vrp(3)+b5;
            if new_vrp(2)<R4(2)
                new_vrp(2)=R4(2);
                new_vrp(3)=R4(3);
            elseif new_vrp(2)>R1(2)
                new_vrp(2)=R1(2);
                new_vrp(3)=R1(3);
            end
        end
    elseif r_vrp(2)>R1(2)
        new_vrp(2)=R1(2);
        new_vrp(3)=(new_vrp(2)-b5)/a5;
        if new_vrp(3)>R1(3)
            new_vrp(3)=R1(3);
            new_vrp(2)=a5*new_vrp(3)+b5;
            if new_vrp(2)>R1(2)
                new_vrp(2)=R1(2);
                new_vrp(3)=R1(3);
            elseif new_vrp(2)<R4(2)
                new_vrp(2)=R4(2);
                new_vrp(3)=R4(3);
            end
        elseif new_vrp(3)<R2(3)
            new_vrp(3)=R2(3);
            new_vrp(2)=a5*new_vrp(3)+b5;
            if new_vrp(2)>R2(2)
                new_vrp(2)=R2(2);
                new_vrp(3)=R2(3);
            elseif new_vrp(2)<R3(2)
                new_vrp(2)=R3(2);
                new_vrp(3)=R3(3);
            end
        end
    elseif r_vrp(3)<R3(3)
        new_vrp(3)=R3(3);
        new_vrp(2)=a5*new_vrp(3)+b5;
        if new_vrp(2)>R2(2)
            new_vrp(2)=R2(2);
            new_vrp(3)=(new_vrp(2)-b5)/a5;
            if new_vrp(3)<R2(3)
                new_vrp(2)=R2(2);
                new_vrp(3)=R2(3);
            elseif new_vrp(3)>R1(3)
                new_vrp(2)=R1(2);
                new_vrp(3)=R1(3);
            end
        elseif new_vrp(2)<R3(2)
            new_vrp(2)=R3(2);
            new_vrp(3)=(new_vrp(2)-b5)/a5;
            if new_vrp(3)<R3(3)
                new_vrp(2)=R3(2);
                new_vrp(3)=R3(3);
            elseif new_vrp(3)>R4(3)
                new_vrp(2)=R4(2);
                new_vrp(3)=R4(3);
            end 
        end
    elseif r_vrp(3)>R1(3)
        new_vrp(3)=R1(3);
        new_vrp(2)=a5*new_vrp(3)+b5;
        if new_vrp(2)>R1(2)
            new_vrp(2)=R1(2);
            new_vrp(3)=(new_vrp(2)-b5)/a5;
            if new_vrp(3)<R2(3)
                new_vrp(2)=R2(2);
                new_vrp(3)=R2(3);
            elseif new_vrp(3)>R1(3)
                new_vrp(2)=R1(2);
                new_vrp(3)=R1(3);
            end 
        elseif new_vrp(2)<R4(2)
            new_vrp(2)=R4(2);
            new_vrp(3)=(new_vrp(2)-b5)/a5;
            if new_vrp(3)<R3(3)
                new_vrp(2)=R3(2);
                new_vrp(3)=R3(3);
            elseif new_vrp(3)>R4(3)
                new_vrp(2)=R4(2);
                new_vrp(3)=R4(3);
            end 
        end
    end 
end

new_vrp_W=RWR*new_vrp+XWR;





% R1=RWR.'*R1+XWR;
% R2=RWR.'*R2+XWR;
% R3=RWR.'*R3+XWR;
% R4=RWR.'*R4+XWR;
% 
% L1=RWR.'*L1+XWR;
% L2=RWR.'*L2+XWR;
% L3=RWR.'*L3+XWR;
% L4=RWR.'*L4+XWR;

R1=RWR*R1+XWR;
R2=RWR*R2+XWR;
R3=RWR*R3+XWR;
R4=RWR*R4+XWR;

L1=RWR*L1+XWR;
L2=RWR*L2+XWR;
L3=RWR*L3+XWR;
L4=RWR*L4+XWR;

== matlab function Control_model_10DOF_fin/10DoF Walker SimMechanics Model/Graphic/Subsystem/MATLAB Function7 ==
  data: R1W output; R2W output; R3W output; R4W output; L1W output; L2W output; L3W output; L4W output; Right_foot_position input; new_vrp output; TWL input; lFoot parameter; dsegment parameter; r_vrp_W input size=3; r_DCM_W input size=3; new_vrp_W output; outside output; cas output
function [R1W,R2W,R3W,R4W,L1W,L2W,L3W,L4W,new_vrp,new_vrp_W,outside,cas]  = support_polygon(Right_foot_position,TWL,lFoot,dsegment,r_vrp_W,r_DCM_W)


Left_foot_position=TWL(1:3,4);
RWL=TWL(1:3,1:3);

R1W=Right_foot_position+RWL.'*[0;-lFoot/2;-dsegment/2];
R2W=Right_foot_position+RWL.'*[0;-lFoot/2;dsegment/2];
R3W=Right_foot_position+RWL.'*[0;lFoot/2;dsegment/2];
R4W=Right_foot_position+RWL.'*[0;lFoot/2;-dsegment/2];

% R1W=Right_foot_position+[1/4;0;-1/4];
% R2W=Right_foot_position+[1/4;0;1/4];
% R3W=Right_foot_position+[-1/4;0;1/4];
% R4W=Right_foot_position+[-1/4;0;-1/4];

L1W=Left_foot_position+RWL.'*[0;-lFoot/2;-dsegment/2];
L2W=Left_foot_position+RWL.'*[0;-lFoot/2;dsegment/2];
L3W=Left_foot_position+RWL.'*[0;lFoot/2;dsegment/2];
L4W=Left_foot_position+RWL.'*[0;lFoot/2;-dsegment/2];

% L1W=Left_foot_position+[1/4;0;-1/4];
% L2W=Left_foot_position+[1/4;0;1/4];
% L3W=Left_foot_position+[-1/4;0;1/4];
% L4W=Left_foot_position+[-1/4;0;-1/4];

R1=RWL*(R1W-Left_foot_position);
R2=RWL*(R2W-Left_foot_position);
R3=RWL*(R3W-Left_foot_position);
R4=RWL*(R4W-Left_foot_position);

L1=RWL*(L1W-Left_foot_position);
L2=RWL*(L2W-Left_foot_position);
L3=RWL*(L3W-Left_foot_position);
L4=RWL*(L4W-Left_foot_position);

r_vrp=RWL*(r_vrp_W-Left_foot_position);
r_DCM=RWL*(r_DCM_W-Left_foot_position);

%Calcul affine line
a1=(L1(2)-R1(2))/(L1(3)-R1(3));
b1=R1(2)-a1*R1(3);

a2=(L2(2)-R2(2))/(L2(3)-R2(3));
b2=R2(2)-a2*R2(3);

a3=(L3(2)-R3(2))/(L3(3)-R3(3));
b3=R3(2)-a3*R3(3);

a4=(L4(2)-R4(2))/(L4(3)-R4(3));
b4=R4(2)-a4*R4(3);

a5=(r_vrp(2)-r_DCM(2))/(r_vrp(3)-r_DCM(3));
b5=r_DCM(2)-a5*r_DCM(3);

outside=1;

if r_vrp(3)>L4(3) && r_vrp(2)<L4(2) && r_vrp(3)<R2(3) && r_vrp(2)>R2(2)
    outside=0;
    if r_vrp(2)<(a1*r_vrp(3)+b1) || r_vrp(2)>(a3*r_vrp(3)+b3)
        outside=1;
    end
end

cas=0;
%         new_vrp(2)=R3(2);
%         new_vrp(3)=(new_vrp(2)-b5)/a5;
%                 new_vrp(3)=(b5-b4)/(a5-a4);
%                 new_vrp(2)=a5*new_vrp(3)+b5;

new_vrp=r_vrp;

if outside==1
    if r_vrp(2)>L4(2)
        cas=1;
        new_vrp(2)=L4(2);
        new_vrp(3)=(new_vrp(2)-b5)/a5;
        if new_vrp(3)<L4(3)
            cas=2;
            new_vrp(3)=L4(3);
            new_vrp(2)=a5*new_vrp(3)+b5;
            if new_vrp(2)<L1(2)
                cas=3;
                new_vrp(2)=L1(2);
                new_vrp(3)=L1(3);
            elseif new_vrp(2)>L4(2)
                cas=4;
                new_vrp(2)=L4(2);
                new_vrp(3)=L4(3);
            end
        elseif new_vrp(3)>L3(3)
            cas=5;
            new_vrp(3)=(b5-b3)/(a3-a5);
            new_vrp(2)=a5*new_vrp(3)+b5;
            if new_vrp(3)<L3(3)
                cas=6;
                new_vrp(2)=L3(2);
                new_vrp(3)=L3(3);
            elseif new_vrp(3)>R3(3)
                cas=7;
                new_vrp(2)=R3(2);
                new_vrp(3)=(new_vrp(2)-b5)/a5;
                if new_vrp(2)>R3(2)
                    cas=8;
                    new_vrp(2)=R3(2);
                    new_vrp(3)=R3(3);
                elseif new_vrp(2)<R2(2)
                    cas=9;
                    new_vrp(2)=R2(2);
                    new_vrp(3)=R2(3);
                end
            end
        end
    elseif r_vrp(2)<R2(2)
        cas=10;
        new_vrp(2)=R2(2);
        new_vrp(3)=(new_vrp(2)-b5)/a5;
        if new_vrp(3)>R2(3)
            cas=11;
            new_vrp(3)=R2(3);
            new_vrp(2)=a5*new_vrp(3)+b5;
            if new_vrp(2)>R3(2)
                cas=12;
                new_vrp(2)=R3(2);
                new_vrp(3)=R3(3);
            elseif new_vrp(2)<R2(2)
                cas=13;
                new_vrp(2)=R2(2);
                new_vrp(3)=R2(3);
            end
        elseif new_vrp(3)<R1(3)
            cas=14;
            new_vrp(3)=(b5-b1)/(a1-a5);
            new_vrp(2)=a5*new_vrp(3)+b5;
            if new_vrp(3)>R1(3)
                cas=15;
                new_vrp(2)=R1(2);
                new_vrp(3)=R1(3);
            elseif new_vrp(3)<L1(3)
                cas=16;
                new_vrp(3)=L1(3);
                new_vrp(2)=a5*new_vrp(3)+b5;
                if new_vrp(2)>L4(2)
                    cas=17;
                    new_vrp(2)=L4(2);
                    new_vrp(3)=L4(3);
                elseif new_vrp(2)<L1(2)
                    cas=18;
                    new_vrp(2)=L1(2);
                    new_vrp(3)=L1(3);
                end
            end
        end
    elseif r_vrp(3)<L4(3) && (r_vrp(2)>R2(2) && r_vrp(2)<L4(2))
        cas=19;
        new_vrp(3)=L4(3);
        new_vrp(2)=a5*new_vrp(3)+b5;
        if new_vrp(2)>L4(2)
            cas=20;
            new_vrp(2)=L4(2);
            new_vrp(3)=L4(3);
        elseif new_vrp(2)<L1(2)
            cas=21;
            new_vrp(3)=(b5-b1)/(a1-a5);
            new_vrp(2)=a5*new_vrp(3)+b5;
            if new_vrp(2)>L1(2)
                cas=22;
                new_vrp(2)=L1(2);
                new_vrp(3)=L1(3);
            elseif new_vrp(2)<R1(2)
                cas=23;
                new_vrp(2)=R1(2);
                new_vrp(3)=R1(3);
            end
        end
    elseif r_vrp(3)>R2(3) && (r_vrp(2)>R2(2) && r_vrp(2)<L4(2))
        cas=24;
        new_vrp(3)=R2(3);
        new_vrp(2)=a5*new_vrp(3)+b5;
        if new_vrp(2)<R2(2)
            cas=25;
            new_vrp(2)=R2(2);
            new_vrp(3)=R2(3);
        elseif new_vrp(2)>R3(2)
            cas=26;
            new_vrp(3)=(b5-b3)/(a3-a5);
            new_vrp(2)=a5*new_vrp(3)+b5;
            if new_vrp(2)<R3(2)
                cas=27;
                new_vrp(2)=R3(2);
                new_vrp(3)=R3(3);
            elseif new_vrp(2)>L3(2)
                cas=28;
                new_vrp(2)=L3(2);
                new_vrp(3)=L3(3);
            end
        end
    elseif r_vrp(2)>a3*r_vrp(3)+b3 && r_vrp(3)<R3(3) && r_vrp(2)<L3(2)
        cas=29;
        new_vrp(3)=(b5-b3)/(a3-a5);
        new_vrp(2)=a5*new_vrp(3)+b5;
        if new_vrp(3)<L3(3)
            cas=30;
            new_vrp(2)=L3(2);
            new_vrp(3)=L3(3);
        elseif new_vrp(2)<R3(2)
            cas=31;
            new_vrp(2)=R3(2);
            new_vrp(3)=R3(3);
        end
    elseif r_vrp(2)<a1*r_vrp(3)+b1 && r_vrp(3)>L1(3) && r_vrp(2)>R1(2)
        cas=32;
        new_vrp(3)=(b5-b1)/(a1-a5);
        new_vrp(2)=a5*new_vrp(3)+b5;
        if new_vrp(2)>L1(2)
            cas=33;
            new_vrp(2)=L1(2);
            new_vrp(3)=L1(3);
        elseif new_vrp(3)>R1(3)
            cas=34;
            new_vrp(2)=R1(2);
            new_vrp(3)=R1(3);
        end
    end
end



new_vrp_W=RWL.'*new_vrp+Left_foot_position;

== matlab function Control_model_10DOF_fin/10DoF Walker SimMechanics Model/Hip AA/MATLAB Function ==
  data: joint input; velocity input; desired_torque input; torque output; validity_angle parameter
function torque = fcn(joint,velocity,desired_torque,validity_angle)

kp=900;
kv=0.008;

min=validity_angle(4,1);
max=validity_angle(4,2);

if joint<=min
    torque=kp*(min-joint)-kv*velocity;
    if torque<=0
        torque=desired_torque;
    end
elseif joint>=max
    torque=kp*(max-joint)-kv*velocity;
    if torque>=0
        torque=desired_torque;
    end
else
    torque=desired_torque;
end

== matlab function Control_model_10DOF_fin/10DoF Walker SimMechanics Model/Hip AA1/MATLAB Function ==
  data: joint input; velocity input; desired_torque input; torque output; validity_angle parameter
function torque = fcn(joint,velocity,desired_torque,validity_angle)

kp=900;
kv=0.008;

min=validity_angle(5,1);
max=validity_angle(5,2);

if joint<=min
    torque=kp*(min-joint)-kv*velocity;
    if torque<=0
        torque=desired_torque;
    end
elseif joint>=max
    torque=kp*(max-joint)-kv*velocity;
    if torque>=0
        torque=desired_torque;
    end
else
    torque=desired_torque;
end

== matlab function Control_model_10DOF_fin/10DoF Walker SimMechanics Model/Hip FE/MATLAB Function ==
  data: joint input; velocity input; desired_torque input; torque output; validity_angle parameter
function torque = fcn(joint,velocity,desired_torque,validity_angle)

kp=900;
kv=0.008;

min=validity_angle(3,1);
max=validity_angle(3,2);

if joint<=min
    torque=kp*(min-joint)-kv*velocity;
    if torque<=0
        torque=desired_torque;
    end
elseif joint>=max
    torque=kp*(max-joint)-kv*velocity;
    if torque>=0
        torque=desired_torque;
    end
else
    torque=desired_torque;
end

== matlab function Control_model_10DOF_fin/10DoF Walker SimMechanics Model/Hip FE1/MATLAB Function ==
  data: joint input; velocity input; desired_torque input; torque output; validity_angle parameter
function torque = fcn(joint,velocity,desired_torque,validity_angle)

kp=900;
kv=0.008;

min=validity_angle(6,1);
max=validity_angle(6,2);

if joint<=min
    torque=kp*(min-joint)-kv*velocity;
    if torque<=0
        torque=desired_torque;
    end
elseif joint>=max
    torque=kp*(max-joint)-kv*velocity;
    if torque>=0
        torque=desired_torque;
    end
else
    torque=desired_torque;
end
